simulink model "Simulink_09_Nov"  (R2020a)
settings: Solver=VariableStepAuto  StartTime=0.0  StopTime=200  RelTol=1e-3
libraries: cstblocks x5
settings Model: Creator=geral  LastModifiedBy=geral

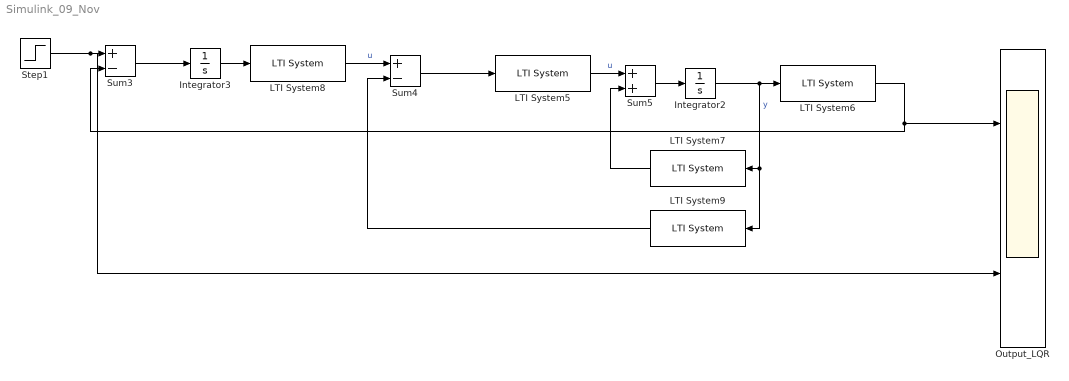
== system Simulink_09_Nov ==
  Integrator2 : Integrator
  Integrator3 : Integrator
  LTI System5 : cstblocks/LTI System  sys=Heli_ss.B  IC=[]
  LTI System6 : cstblocks/LTI System  sys=[1 0 0 0]  IC=[]
  LTI System7 : cstblocks/LTI System  sys=Heli_ss.A  IC=[]
  LTI System8 : cstblocks/LTI System  sys=Ki_LQR  IC=[]
  LTI System9 : cstblocks/LTI System  sys=K_LQR  IC=[]
  Output_LQR : Scope  NumInputPorts=2
  Step1 : Step  Time=0.1  After=10  SampleTime=0
  Sum3 : Sum  Inputs=+-
  Sum4 : Sum  Inputs=+-
  Sum5 : Sum
  wires:
  LTI System5/1 -> Sum5/1  "u"
  Integrator3/1 -> LTI System8/1
  LTI System7/1 -> Sum5/2
  LTI System8/1 -> Sum4/1  "u"
  Step1/1 -> Output_LQR/2, Sum3/1
  LTI System6/1 -> Sum3/2, Output_LQR/1
  Sum3/1 -> Integrator3/1
  Integrator2/1 -> LTI System6/1, LTI System9/1, LTI System7/1  "y"
  Sum5/1 -> Integrator2/1
  LTI System9/1 -> Sum4/2
  Sum4/1 -> LTI System5/1
